simulink library "scarsLibrary"  (R2019b)
settings: Solver=VariableStepAuto  StartTime=0.0  StopTime=10.0  RelTol=1e-3
undefined symbols (not defined in the file): A_x, A_y, A_z, Actuators, added_noise, axis_switch, bb, C_d, decsec, decstart, delay, Detumbling, displacement, Earth, IAU, initDay, initEuler, initYear, linsys1, mag_sat, Magnetorquers, multiplied_noise, Re, rw, scars_library, st_freq, startTime, sun_position, t_power, WGS84
libraries: $bdroot x89, aerolibutil x15, sharedtransform x12, vrlib x9, simulink x6, aerolibtransform2 x2, aerolibgravity2 x2, aerolib6dof2 x2, simulink_extras x2, aerolibatmos2 x1, aerolibnav x1
(part 2 of 2)

== system scarsLibrary/PW-Sat2/Environment ==
  SatStates : Inport
  Atmosphere [kg/m^3] : $bdroot/Environment/Atmosphere [kg//m^3]  SystemSampleTime=-1  Latency=0  AutoFrameSizeCalculation=off
  Atmospheric Drag [N]1 : $bdroot/Environment/Atmospheric Drag [N]  SystemSampleTime=-1  Latency=0  AutoFrameSizeCalculation=off
      link override Drag [N]/Constant1: Value=area_vector
  Bus Creator : BusCreator  Inputs=4
  Gravity [N]1 : $bdroot/Environment/Gravity [N]  mass=1
  Ground : Ground
  Magnetic Field [nT]1 : $bdroot/Environment/Magnetic Field [nT]  SystemSampleTime=-1  Latency=0  AutoFrameSizeCalculation=off
  Scope : Scope
  Sum : Sum  Inputs=+|+
  Sun's Position [km]1 : $bdroot/Environment/Sun's Position [km]  SystemSampleTime=-1  Latency=0  AutoFrameSizeCalculation=off
  Env : Outport
  Forces : Outport  Port=2
  Moments : Outport  Port=3
  wires:
  Ground/1 -> Moments/1
  Atmosphere [kg/m^3]/1 -> Bus Creator/4  "Atmosphere Density [kg/m^3]"
  Gravity [N]1/1 -> Sum/2
  Bus Creator/1 -> Env/1
  Atmospheric Drag [N]1/1 -> Scope/1, Sum/1
  Magnetic Field [nT]1/1 -> Bus Creator/1  "Magnetic Field [nT]"
  Sun's Position [km]1/1 -> Bus Creator/3  "Sun's Position [km]"
  Sum/1 -> Forces/1, Bus Creator/2  "Environment Force [N]"
  SatStates/1 -> Gravity [N]1/1, Atmosphere [kg/m^3]/1, Atmospheric Drag [N]1/1, Magnetic Field [nT]1/1

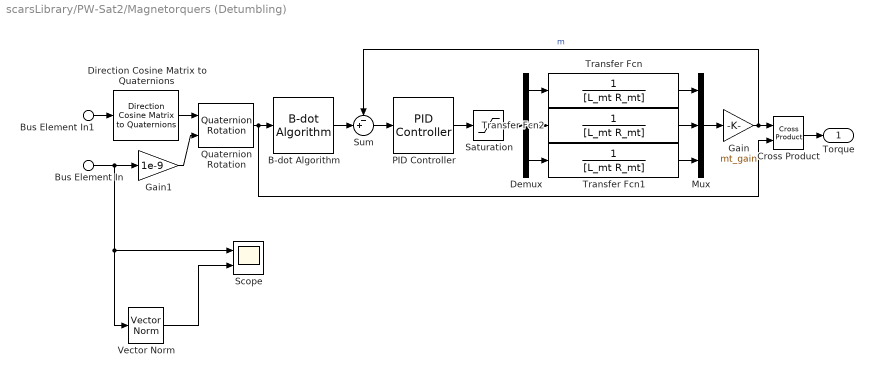
== system scarsLibrary/PW-Sat2/Magnetorquers (Detumbling) ==
  Bus Element In : Inport  PortName=Env  Element=Magnetic Field [nT]
  Bus Element In1 : Inport  Port=2  PortName=SatStates  Element=DCM_NED2B
  B-dot Algorithm : $bdroot/ Control Algorithms /B-dot Algorithm  k_gain=-0.1
  Cross Product : vrlib/Utilities/Cross Product
      settings: SourceProductName=Simulink
  Demux : Demux  Outputs=3
  Direction Cosine Matrix to Quaternions : sharedtransform/Direction Cosine Matrix  to Quaternions  aMode=0  action=None  tolerance=eps(2)
      settings: SourceProductName=Aerospace Blockset  SourceProductBaseCode=AE
  Gain : Gain  Gain=mt_gain
  Gain1 : Gain  Gain=1e-9
  Mux : Mux  Inputs=3
  PID Controller : $bdroot/ Control Algorithms /PID Controller  Kp=1  Ki=0  Kd=0  pid_sat_max=inf  pid_sat_min=-inf  pid_dz_max=0  pid_dz_min=0
  Quaternion Rotation : aerolibutil/Quaternion Rotation
  Saturation : Saturate  UpperLimit=mag_sat  LowerLimit=-mag_sat
  Scope : Scope  NumInputPorts=2
  Sum : Sum  Inputs=-+|
  Transfer Fcn : TransferFcn  Denominator=[L_mt R_mt]
  Transfer Fcn1 : TransferFcn  Denominator=[L_mt R_mt]
  Transfer Fcn2 : TransferFcn  Denominator=[L_mt R_mt]
  Vector Norm : $bdroot/Vector Norm  SystemSampleTime=-1  Latency=0  AutoFrameSizeCalculation=off
  Torque : Outport
  wires:
  Gain1/1 -> Quaternion Rotation/2
  Gain/1 -> Cross Product/1, Sum/1  "m"
  Bus Element In1/1 -> Direction Cosine Matrix to Quaternions/1
  Transfer Fcn2/1 -> Mux/2
  Cross Product/1 -> Torque/1
  Transfer Fcn1/1 -> Mux/3
  Bus Element In/1 -> Vector Norm/1, Scope/1, Gain1/1
  Transfer Fcn/1 -> Mux/1
  Demux/2 -> Transfer Fcn2/1
  Mux/1 -> Gain/1
  Quaternion Rotation/1 -> B-dot Algorithm/1, Cross Product/2
  Direction Cosine Matrix to Quaternions/1 -> Quaternion Rotation/1
  Sum/1 -> PID Controller/1
  Saturation/1 -> Demux/1
  Demux/1 -> Transfer Fcn/1
  B-dot Algorithm/1 -> Sum/2
  Demux/3 -> Transfer Fcn1/1
  PID Controller/1 -> Saturation/1
  Vector Norm/1 -> Scope/2

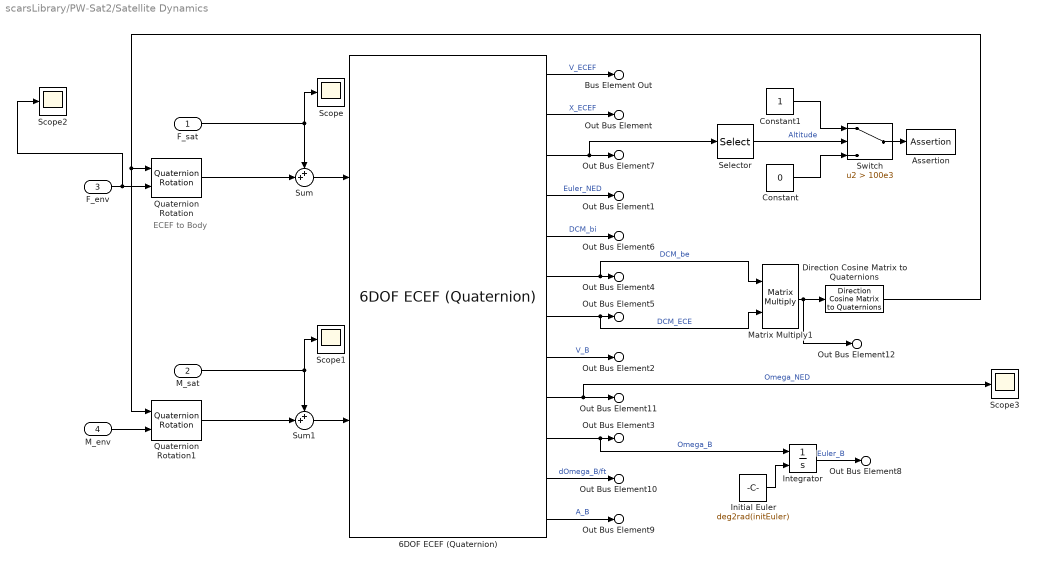
== system scarsLibrary/PW-Sat2/Satellite Dynamics ==
  note: ECEF to Body
  F_sat : Inport
  M_sat : Inport  Port=2
  F_env : Inport  Port=3
  M_env : Inport  Port=4
  6DOF ECEF (Quaternion) : aerolib6dof2/6DOF ECEF (Quaternion)  units=Metric (MKS)  mtype=Fixed  xg_0=r_lla  Vm_0=v_b  eul_0=deg2rad(initEuler)  pm_0=[0.1 0.2 0.3]  mass_0=1  mass_e=0.5  mass_f=2.0  inertia=eye(3)  inertia_e=eye(3)  inertia_f=2*eye(3)  vre_flag=on  abi_flag=off  ptype=Earth (WGS84)  R=6378137  F=1/298.257223563  w_E=7292115e-11  angle_in=Internal  LG0=0  quat_statename=''  pm_statename=''  Vm_statename=''  posECEF_statename=''  posECI_statename=''  LG_statename=''  mass_statename=''
      settings: SourceProductName=Aerospace Blockset  SourceProductBaseCode=AE
  Assertion : Assertion
  Constant : Constant  Value=0
  Constant1 : Constant
  Direction Cosine Matrix to Quaternions : sharedtransform/Direction Cosine Matrix  to Quaternions  aMode=0  action=None  tolerance=eps(2)
      settings: SourceProductName=Aerospace Blockset  SourceProductBaseCode=AE
  Initial Euler : Constant  Value=deg2rad(initEuler)
  Integrator : Integrator  InitialConditionSource=external  WrapState=on
  Matrix Multiply1 : Product  Multiplication=Matrix(*)
  Quaternion Rotation : aerolibutil/Quaternion Rotation
  Quaternion Rotation1 : aerolibutil/Quaternion Rotation
  Scope{,1..3} (4 alike) : Scope
  Selector : Selector  InputPortWidth=3  IndexOptions=Index vector (dialog)  Indices=3  OutputSizes=1
  Sum : Sum  Inputs=++|
  Sum1 : Sum  Inputs=++|
  Switch : Switch  Criteria=u2 > Threshold  Threshold=100e3
  Bus Element Out : Outport  PortName=SatStates  Element=V_ECEF
  Out Bus Element : Outport  PortName=SatStates  Element=X_ECEF
  Out Bus Element1 : Outport  PortName=SatStates  Element=Euler_NED
  Out Bus Element2 : Outport  PortName=SatStates  Element=V_B
  Out Bus Element3 : Outport  PortName=SatStates  Element=Omega_B
  Out Bus Element6 : Outport  PortName=SatStates  Element=DCM_ECI2B
  Out Bus Element4 : Outport  PortName=SatStates  Element=DCM_NED2B
  Out Bus Element5 : Outport  PortName=SatStates  Element=DCM_ECEF2NED
  Out Bus Element7 : Outport  PortName=SatStates  Element=lla
  Out Bus Element8 : Outport  PortName=SatStates  Element=Euler_B
  Out Bus Element9 : Outport  PortName=SatStates  Element=A_B
  Out Bus Element10 : Outport  PortName=SatStates  Element=dOmega_B/dt
  Out Bus Element11 : Outport  PortName=SatStates  Element=Omega_NED
  Out Bus Element12 : Outport  PortName=SatStates  Element=DCM_ECEF2B
  wires:
  Constant/1 -> Switch/3
  6DOF ECEF (Quaternion)/9 -> Scope3/1, Out Bus Element11/1  "Omega_NED"
  Initial Euler/1 -> Integrator/2
  M_env/1 -> Quaternion Rotation1/2
  6DOF ECEF (Quaternion)/12 -> Out Bus Element9/1  "A_B"
  6DOF ECEF (Quaternion)/7 -> Matrix Multiply1/2, Out Bus Element5/1  "DCM_ECE"
  6DOF ECEF (Quaternion)/11 -> Out Bus Element10/1  "dOmega_B/ft"
  6DOF ECEF (Quaternion)/3 -> Selector/1, Out Bus Element7/1
  6DOF ECEF (Quaternion)/5 -> Out Bus Element6/1  "DCM_bi"
  Sum/1 -> 6DOF ECEF (Quaternion)/1
  Integrator/1 -> Out Bus Element8/1  "Euler_B"
  Direction Cosine Matrix to Quaternions/1 -> Quaternion Rotation1/1, Quaternion Rotation/1
  F_sat/1 -> Scope/1, Sum/1
  Quaternion Rotation/1 -> Sum/2
  Quaternion Rotation1/1 -> Sum1/2
  Sum1/1 -> 6DOF ECEF (Quaternion)/2
  Matrix Multiply1/1 -> Direction Cosine Matrix to Quaternions/1, Out Bus Element12/1
  6DOF ECEF (Quaternion)/1 -> Bus Element Out/1  "V_ECEF"
  Selector/1 -> Switch/2  "Altitude"
  6DOF ECEF (Quaternion)/4 -> Out Bus Element1/1  "Euler_NED"
  6DOF ECEF (Quaternion)/6 -> Matrix Multiply1/1, Out Bus Element4/1  "DCM_be"
  6DOF ECEF (Quaternion)/2 -> Out Bus Element/1  "X_ECEF"
  Switch/1 -> Assertion/1
  Constant1/1 -> Switch/1
  6DOF ECEF (Quaternion)/10 -> Integrator/1, Out Bus Element3/1  "Omega_B"
  6DOF ECEF (Quaternion)/8 -> Out Bus Element2/1  "V_B"
  M_sat/1 -> Sum1/1, Scope1/1
  F_env/1 -> Scope2/1, Quaternion Rotation/2

== system scarsLibrary/Sensors/Accelerometer ==
  SatStates : Inport
  Bus Element In : Inport  Port=2  PortName=Env  Element=Gravitational Force [N]
  Bus Selector : BusSelector  OutputSignals=A_B,Omega_B,dOmega_B/dt
  Constant : Constant  Value=[0 0 0]
  Three-axis Accelerometer : aerolibnav/Three-axis Accelerometer  units=Metric (MKS)  acc=acc  gtype=on  dtype_a=on  w_a=w_a  z_a=z_a  a_sf_cc=[1 0 0; 0 1 0; 0 0 1]  a_bias=a_bias*[1 1 1]  a_Ts=0  a_rand=on  a_seeds=[23093 23094 23095]  a_pow=a_pow*[1 1 1]  a_sat="[-a_min  -a_min  -a_min a_max a_max a_max]"
      settings: SourceProductName=Aerospace Blockset  SourceProductBaseCode=AE
  Zero-Order Hold : ZeroOrderHold  SampleTime=1/freq
  A_B : Outport
  wires:
  SatStates/1 -> Bus Selector/1
  Constant/1 -> Three-axis Accelerometer/4
  Bus Selector/1 -> Three-axis Accelerometer/1  "<A_B>"
  Bus Selector/2 -> Three-axis Accelerometer/2  "<Omega_B>"
  Bus Selector/3 -> Three-axis Accelerometer/3  "<dOmega_B/dt>"
  Bus Element In/1 -> Three-axis Accelerometer/5
  Three-axis Accelerometer/1 -> Zero-Order Hold/1
  Zero-Order Hold/1 -> A_B/1

== system scarsLibrary/Sensors/Earth- & Sun-sensor ==
  Bus Element In1 : Inport  PortName=SatStates  Element=X_ECEF
  Bus Element In : Inport  Port=2  PortName=Env  Element=Sun's Position [km]
  Euler_B : Outport
  wires:
  Bus Element In/1 -> Euler_B/1

== system scarsLibrary/Sensors/GPS Receiver ==
  Bus Element In : Inport  PortName=SatStates  Element=X_ECEF
  X_ECEF : Outport
  wires:
  Bus Element In/1 -> X_ECEF/1

== system scarsLibrary/Sensors/Gyros ==
  note: noise_power  = [0.1]
      | sample_time = 0.1
  note: wn = 1000*2*pi; % natural frequency [not in Hz, but can be transferred] dynamics rad/s
      | w = 12.5*2*pi; % cutoff frequency [Hz*2pi = deg/s] LPF rad/s
      | zeta = sqrt(2)/2; % damping ratio
      | z = zeta; %?
  Bus Element In : Inport  PortName=SatStates  Element=Omega_B
  Add : Sum
  Add1 : Sum
  Band-Limited White Noise : simulink/Sources/Band-Limited White Noise  Cov=[g_power]  Ts=1/g_freq  seed=[23341]
  Constant : Constant  Value=g_bias
  Demux : Demux  Outputs=3
  Mux : Mux  Inputs=3
  Transfer Fcn : TransferFcn  Numerator=[g_wn^2]  Denominator=[1 2*g_zeta*(g_wn) (g_wn)^2]
  Transfer Fcn1 : TransferFcn  Numerator=[g_wn^2]  Denominator=[1 2*g_zeta*(g_wn) (g_wn)^2]
  Transfer Fcn2 : TransferFcn  Numerator=[g_wn^2]  Denominator=[1 2*g_zeta*(g_wn) (g_wn)^2]
  Zero-Order Hold : ZeroOrderHold  SampleTime=1/g_freq
  Omega_B : Outport
  wires:
  Constant/1 -> Add/2
  Add/1 -> Add1/1
  Band-Limited White Noise/1 -> Add1/2
  Add1/1 -> Zero-Order Hold/1
  Zero-Order Hold/1 -> Omega_B/1
  Bus Element In/1 -> Demux/1
  Demux/2 -> Transfer Fcn/1
  Demux/1 -> Transfer Fcn1/1
  Demux/3 -> Transfer Fcn2/1
  Transfer Fcn/1 -> Mux/2
  Transfer Fcn1/1 -> Mux/1
  Transfer Fcn2/1 -> Mux/3
  Mux/1 -> Add/1

== system scarsLibrary/Sensors/Ideal Angle ==
  Bus Element In : Inport  PortName=SatStates  Element=Euler_B
  Euler_B : Outport
  wires:
  Bus Element In/1 -> Euler_B/1

== system scarsLibrary/Sensors/Ideal Position ==
  Bus Element In : Inport  PortName=SatStates  Element=X_ECEF
  X_ECEF : Outport
  wires:
  Bus Element In/1 -> X_ECEF/1

== system scarsLibrary/Sensors/Ideal Rate ==
  Bus Element In : Inport  PortName=SatStates  Element=Euler_B
  Omega_B : Outport
  wires:
  Bus Element In/1 -> Omega_B/1

== system scarsLibrary/Sensors/Magnetometer ==
  Bus Element In : Inport  PortName=Env  Element=Magnetic Field [nT]
  Bias : Constant  Value=m_bias
  Noise : simulink/Sources/Band-Limited White Noise  Cov=m_power*[1 1 1]  Ts=1/m_freq  seed="[ randi(1000, 1, 3)  ]"
  Sum1 : Sum  Inputs=+++
  "Zero-Order Hold " : ZeroOrderHold  SampleTime=1/m_freq
  B : Outport
  wires:
  Bias/1 -> Sum1/3
  Bus Element In/1 -> Sum1/2
  "Zero-Order Hold "/1 -> B/1
  Noise/1 -> Sum1/1
  Sum1/1 -> "Zero-Order Hold "/1

== system scarsLibrary/Sensors/Simple Angle ==
  Bus Element In : Inport  PortName=SatStates  Element=Euler_B
  Euler_B : Outport
  wires:
  Bus Element In/1 -> Euler_B/1

== system scarsLibrary/Sensors/Simple Position ==
  Bus Element In : Inport  PortName=SatStates  Element=X_ECEF
  X_ECEF : Outport
  wires:
  Bus Element In/1 -> X_ECEF/1

== system scarsLibrary/Sensors/Simple Rate ==
  Bus Element In : Inport  PortName=SatStates  Element=Euler_B
  Omega_B : Outport
  wires:
  Bus Element In/1 -> Omega_B/1

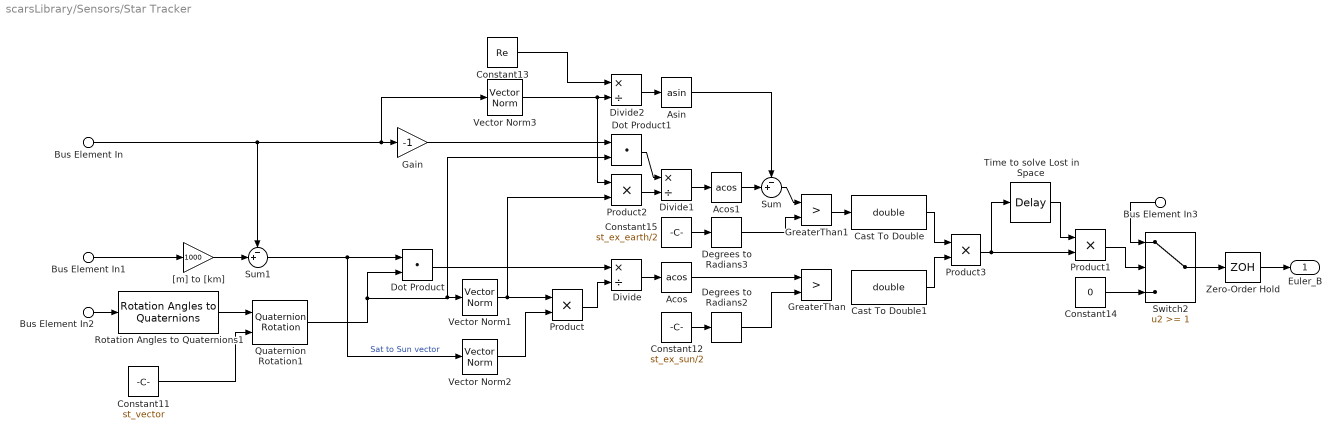
== system scarsLibrary/Sensors/Star Tracker ==
  Bus Element In : Inport  PortName=SatStates  Element=X_ECEF
  Bus Element In2 : Inport  PortName=SatStates  Element=Euler_B
  Bus Element In3 : Inport  PortName=SatStates  Element=Euler_B
  Bus Element In1 : Inport  Port=2  PortName=Env  Element=Sun's Position [km]
  Acos : Trigonometry  Operator=acos
  Acos1 : Trigonometry  Operator=acos
  Asin : Trigonometry  Operator=asin
  Cast To Double : DataTypeConversion  OutDataTypeStr=double
  Cast To Double1 : DataTypeConversion  OutDataTypeStr=double
  Constant11 : Constant  Value=st_vector
  Constant12 : Constant  Value=st_ex_sun/2
  Constant13 : Constant  Value=Re
  Constant14 : Constant  Value=0
  Constant15 : Constant  Value=st_ex_earth/2
  Degrees to Radians2 : simulink_extras/Transformations/Degrees to Radians
  Degrees to Radians3 : simulink_extras/Transformations/Degrees to Radians
  Divide : Product  Inputs=*/
  Divide1 : Product  Inputs=*/
  Divide2 : Product  Inputs=*/
  Dot Product : DotProduct  InputSameDT=on  OutDataTypeStr=Inherit: Inherit via internal rule
  Dot Product1 : DotProduct  InputSameDT=on  OutDataTypeStr=Inherit: Inherit via internal rule
  Gain : Gain  Gain=-1
  GreaterThan : RelationalOperator  Operator=>  OutDataTypeStr=boolean  RndMeth=Simplest
  GreaterThan1 : RelationalOperator  Operator=>  OutDataTypeStr=boolean  RndMeth=Simplest
  Product{,1..3} (4 alike) : Product
  Quaternion Rotation1 : aerolibutil/Quaternion Rotation
  Rotation Angles to Quaternions1 : sharedtransform/Rotation Angles to Quaternions  rotationOrder=XYZ  aMode=aMode
      settings: SourceProductName=Aerospace Blockset  SourceProductBaseCode=AE
  Sum : Sum  Inputs=-+|
  Sum1 : Sum  Inputs=-+|
  Switch2 : Switch  Threshold=1
  Time to solve Lost in Space : TransportDelay  DelayTime=st_lost  InitialOutput=1
  Vector Norm1 : $bdroot/Vector Norm  SystemSampleTime=-1  Latency=0  AutoFrameSizeCalculation=off
  Vector Norm2 : $bdroot/Vector Norm  SystemSampleTime=-1  Latency=0  AutoFrameSizeCalculation=off
  Vector Norm3 : $bdroot/Vector Norm  SystemSampleTime=-1  Latency=0  AutoFrameSizeCalculation=off
  Zero-Order Hold : ZeroOrderHold  SampleTime=1/st_freq
  "[m] to [km]" : Gain  Gain=1000
  Euler_B : Outport
  wires:
  Rotation Angles to Quaternions1/1 -> Quaternion Rotation1/1
  Bus Element In/1 -> Sum1/1, Vector Norm3/1, Gain/1
  Acos/1 -> GreaterThan/1
  Constant13/1 -> Divide2/1
  "[m] to [km]"/1 -> Sum1/2
  Quaternion Rotation1/1 -> Dot Product/2, Dot Product1/2, Vector Norm1/1
  Vector Norm1/1 -> Product2/2, Product/1
  Product/1 -> Divide/2
  Switch2/1 -> Zero-Order Hold/1
  Bus Element In2/1 -> Rotation Angles to Quaternions1/1
  Product1/1 -> Switch2/2
  Product3/1 -> Time to solve Lost in Space/1, Product1/2
  Constant15/1 -> Degrees to Radians3/1
  Degrees to Radians3/1 -> GreaterThan1/2
  Constant14/1 -> Switch2/3
  Vector Norm3/1 -> Product2/1, Divide2/2
  Time to solve Lost in Space/1 -> Product1/1
  Sum1/1 -> Vector Norm2/1, Dot Product/1  "Sat to Sun vector"
  Degrees to Radians2/1 -> GreaterThan/2
  Product2/1 -> Divide1/2
  Dot Product/1 -> Divide/1
  Constant11/1 -> Quaternion Rotation1/2
  Divide2/1 -> Asin/1
  Bus Element In3/1 -> Switch2/1
  Constant12/1 -> Degrees to Radians2/1
  Dot Product1/1 -> Divide1/1
  Gain/1 -> Dot Product1/1
  Divide1/1 -> Acos1/1
  Divide/1 -> Acos/1
  Bus Element In1/1 -> "[m] to [km]"/1
  Vector Norm2/1 -> Product/2
  Acos1/1 -> Sum/2
  Sum/1 -> GreaterThan1/1
  Asin/1 -> Sum/1
  Zero-Order Hold/1 -> Euler_B/1
  GreaterThan1/1 -> Cast To Double/1
  Cast To Double1/1 -> Product3/2
  Cast To Double/1 -> Product3/1

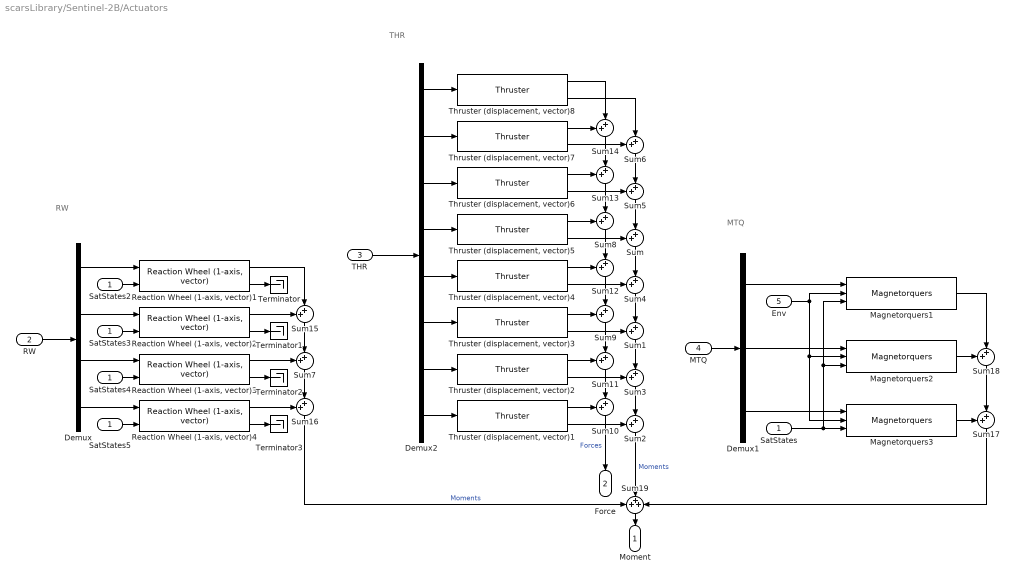
== system scarsLibrary/Sentinel-2B/Actuators ==
  note: MTQ
  note: RW
  note: THR
  SatStates : Inport
  RW : Inport  Port=2
  THR : Inport  Port=3
  MTQ : Inport  Port=4
  Env : Inport  Port=5
  Demux : Demux
  Demux1 : Demux  Outputs=3
  Demux2 : Demux  Outputs=8
  Magnetorquers1 : $bdroot/Actuators/Magnetorquers  L_mt=2.666  R_mt=3.621  l_c_mt=0.25  w_c_mt=7.965e-3  d_w_mt=4.04e-4  mag_vol_max=3  mag_vol_min=-3
  Magnetorquers2 : $bdroot/Actuators/Magnetorquers  L_mt=2.666  R_mt=3.621  l_c_mt=0.25  w_c_mt=7.965e-3  d_w_mt=4.04e-4  mag_vol_max=3  mag_vol_min=-3
  Magnetorquers3 : $bdroot/Actuators/Magnetorquers  L_mt=2.666  R_mt=3.621  l_c_mt=0.25  w_c_mt=7.965e-3  d_w_mt=4.04e-4  mag_vol_max=3  mag_vol_min=-3
  Reaction Wheel (1-axis, vector){1..4} (4 alike) : $bdroot/Actuators/Reaction Wheel (1-axis, vector)  op_vect=[1 1 1]  N=25e-3  R=0.1  J=1  c=0.0001  vel_max=6000*2*pi/60  torq_max=1.5e-3  i_max=0.5  rw_power=0.0001  rw_freq=0.1
  SatStates{2..5} (4 alike) : InportShadow
  Sum{,1..18} (19 alike) : Sum  Inputs=++|
  Sum19 : Sum  Inputs=+++
  Terminator{,1..3} (4 alike) : Terminator
  Thruster (displacement, vector){1..8} (8 alike) : $bdroot/Actuators/Thruster  SystemSampleTime=-1  Latency=0  AutoFrameSizeCalculation=off
  Moment : Outport
  Force : Outport  Port=2
  wires:
  Demux2/1 -> "Thruster (displacement, vector)8"/1
  "Reaction Wheel (1-axis, vector)4"/1 -> Sum16/1
  Sum15/1 -> Sum7/2
  Demux/4 -> "Reaction Wheel (1-axis, vector)4"/1
  "Thruster (displacement, vector)2"/2 -> Sum3/1
  "Thruster (displacement, vector)2"/1 -> Sum11/1
  "Thruster (displacement, vector)3"/2 -> Sum1/1
  Sum6/1 -> Sum5/2
  "Thruster (displacement, vector)6"/2 -> Sum5/1
  "Reaction Wheel (1-axis, vector)4"/2 -> Terminator3/1
  Demux2/3 -> "Thruster (displacement, vector)6"/1
  Sum13/1 -> Sum8/2
  Demux1/3 -> Magnetorquers3/1
  Sum11/1 -> Sum10/2
  Sum14/1 -> Sum13/2
  "Thruster (displacement, vector)7"/2 -> Sum6/1
  Sum/1 -> Sum4/2
  Sum9/1 -> Sum11/2
  Sum8/1 -> Sum12/2
  "Thruster (displacement, vector)7"/1 -> Sum14/1
  Demux1/2 -> Magnetorquers2/1
  Sum2/1 -> Sum19/2  "Moments"
  Demux2/5 -> "Thruster (displacement, vector)4"/1
  Demux1/1 -> Magnetorquers1/1
  "Thruster (displacement, vector)4"/2 -> Sum4/1
  Sum4/1 -> Sum1/2
  "Reaction Wheel (1-axis, vector)2"/1 -> Sum15/1
  Env/1 -> Magnetorquers1/2, Magnetorquers3/2, Magnetorquers2/2
  Demux/2 -> "Reaction Wheel (1-axis, vector)2"/1
  Sum10/1 -> Force/1  "Forces"
  Sum16/1 -> Sum19/1  "Moments"
  Demux2/2 -> "Thruster (displacement, vector)7"/1
  SatStates/1 -> Magnetorquers1/3, Magnetorquers2/3, Magnetorquers3/3
  "Reaction Wheel (1-axis, vector)1"/2 -> Terminator/1
  "Reaction Wheel (1-axis, vector)3"/2 -> Terminator2/1
  Sum5/1 -> Sum/2
  "Reaction Wheel (1-axis, vector)2"/2 -> Terminator1/1
  Demux2/8 -> "Thruster (displacement, vector)1"/1
  "Thruster (displacement, vector)8"/2 -> Sum6/2
  SatStates3/1 -> "Reaction Wheel (1-axis, vector)2"/2
  SatStates5/1 -> "Reaction Wheel (1-axis, vector)4"/2
  Demux/3 -> "Reaction Wheel (1-axis, vector)3"/1
  SatStates4/1 -> "Reaction Wheel (1-axis, vector)3"/2
  Demux2/7 -> "Thruster (displacement, vector)2"/1
  Demux2/6 -> "Thruster (displacement, vector)3"/1
  Demux/1 -> "Reaction Wheel (1-axis, vector)1"/1
  Sum1/1 -> Sum3/2
  "Reaction Wheel (1-axis, vector)1"/1 -> Sum15/2
  "Thruster (displacement, vector)4"/1 -> Sum12/1
  Demux2/4 -> "Thruster (displacement, vector)5"/1
  Sum7/1 -> Sum16/2
  "Thruster (displacement, vector)6"/1 -> Sum13/1
  "Thruster (displacement, vector)1"/2 -> Sum2/1
  "Thruster (displacement, vector)1"/1 -> Sum10/1
  "Thruster (displacement, vector)5"/2 -> Sum/1
  Sum3/1 -> Sum2/2
  "Reaction Wheel (1-axis, vector)3"/1 -> Sum7/1
  SatStates2/1 -> "Reaction Wheel (1-axis, vector)1"/2
  "Thruster (displacement, vector)5"/1 -> Sum8/1
  "Thruster (displacement, vector)8"/1 -> Sum14/2
  Sum12/1 -> Sum9/2
  "Thruster (displacement, vector)3"/1 -> Sum9/1
  Sum18/1 -> Sum17/2
  Sum17/1 -> Sum19/3
  Magnetorquers1/1 -> Sum18/2
  Magnetorquers2/1 -> Sum18/1
  Magnetorquers3/1 -> Sum17/1
  Sum19/1 -> Moment/1
  RW/1 -> Demux/1
  THR/1 -> Demux2/1
  MTQ/1 -> Demux1/1

== system scarsLibrary/Sentinel-2B/OBC ==
  Sensors : Inport
  Ground : Ground
  Ground1 : Ground
  Ground2 : Ground
  Terminator : Terminator
  RW : Outport
  THR : Outport  Port=2
  MTQ : Outport  Port=3
  wires:
  Sensors/1 -> Terminator/1
  Ground/1 -> RW/1
  Ground1/1 -> THR/1
  Ground2/1 -> MTQ/1

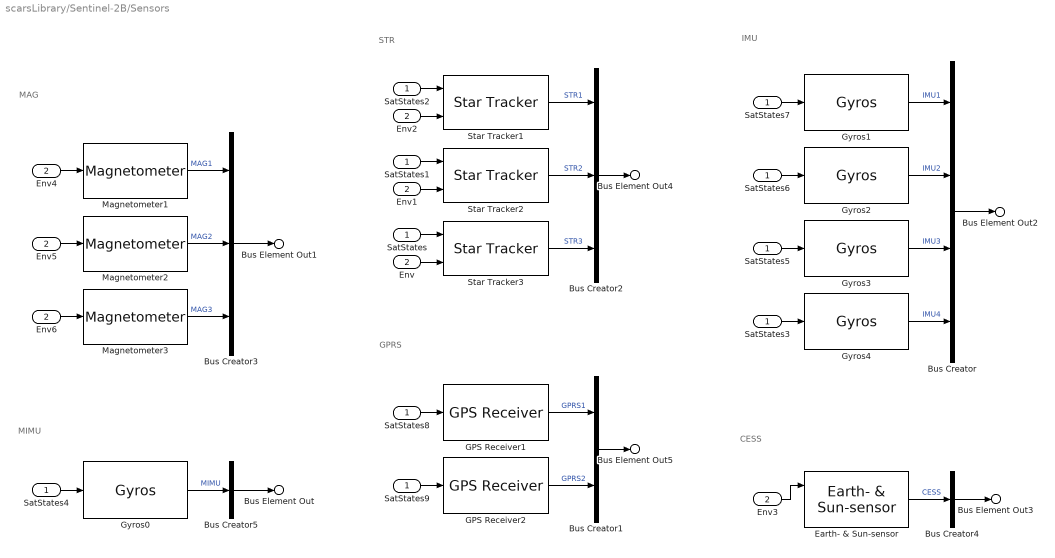
== system scarsLibrary/Sentinel-2B/Sensors ==
  note: MIMU
  note: MAG
  note: CESS
  note: IMU
  note: GPRS
  note: STR
  "SatStates " : Inport
  "Env " : Inport  Port=2
  Bus Creator : BusCreator  Inputs=4
  Bus Creator1 : BusCreator  Inputs=2
  Bus Creator2 : BusCreator  Inputs=3
  Bus Creator3 : BusCreator  Inputs=3
  Bus Creator4 : BusCreator  Inputs=1
  Bus Creator5 : BusCreator  Inputs=1
  Earth- & Sun-sensor : $bdroot/Sensors/Earth- & Sun-sensor  SystemSampleTime=-1  Latency=0  AutoFrameSizeCalculation=off
  Env{1..6} (6 alike) : InportShadow  Port=2
  GPS Receiver1 : $bdroot/Sensors/GPS Receiver  SystemSampleTime=-1  Latency=0  AutoFrameSizeCalculation=off
  GPS Receiver2 : $bdroot/Sensors/GPS Receiver  SystemSampleTime=-1  Latency=0  AutoFrameSizeCalculation=off
  Gyros{0..4} (5 alike) : $bdroot/Sensors/Gyros  g_wn=1000*2*pi  g_zeta=sqrt(2)/2  g_freq=80  g_bias=0  g_power=(0.04)^2  g_max=deg2rad(100)  g_min=-deg2rad(100)
  Magnetometer1 : $bdroot/Sensors/Magnetometer  m_power=0.1  m_freq=10  m_bias=[0.01 0.01 0.01]
  Magnetometer2 : $bdroot/Sensors/Magnetometer  m_power=0.1  m_freq=10  m_bias=[0.01 0.01 0.01]
  Magnetometer3 : $bdroot/Sensors/Magnetometer  m_power=0.1  m_freq=10  m_bias=[0.01 0.01 0.01]
  SatStates{1..9} (9 alike) : InportShadow
  Star Tracker1 : $bdroot/Sensors/Star Tracker  st_vector=[0 0 -1]  st_ex_sun=20  st_ex_earth=20  st_lost=5  Parameter5=10
  Star Tracker2 : $bdroot/Sensors/Star Tracker  st_vector=[0 0 -1]  st_ex_sun=20  st_ex_earth=20  st_lost=5  Parameter5=10
  Star Tracker3 : $bdroot/Sensors/Star Tracker  st_vector=[0 0 -1]  st_ex_sun=20  st_ex_earth=20  st_lost=5  Parameter5=10
  Bus Element Out : Outport  PortName=Sensors  Element=MIMU
  Bus Element Out1 : Outport  PortName=Sensors  Element=MAG
  Bus Element Out2 : Outport  PortName=Sensors  Element=IMU
  Bus Element Out3 : Outport  PortName=Sensors  Element=CESS
  Bus Element Out4 : Outport  PortName=Sensors  Element=STR
  Bus Element Out5 : Outport  PortName=Sensors  Element=GPRS
  wires:
  Env1/1 -> Star Tracker2/2
  Star Tracker1/1 -> Bus Creator2/1  "STR1"
  SatStates1/1 -> Star Tracker2/1
  Star Tracker2/1 -> Bus Creator2/2  "STR2"
  Env2/1 -> Star Tracker1/2
  "Env "/1 -> Star Tracker3/2
  "SatStates "/1 -> Star Tracker3/1
  Star Tracker3/1 -> Bus Creator2/3  "STR3"
  SatStates2/1 -> Star Tracker1/1
  Env5/1 -> Magnetometer2/1
  Env4/1 -> Magnetometer1/1
  Magnetometer1/1 -> Bus Creator3/1  "MAG1"
  Env6/1 -> Magnetometer3/1
  Magnetometer2/1 -> Bus Creator3/2  "MAG2"
  SatStates8/1 -> GPS Receiver1/1
  Env3/1 -> Earth- & Sun-sensor/1
  SatStates9/1 -> GPS Receiver2/1
  GPS Receiver2/1 -> Bus Creator1/2  "GPRS2"
  Magnetometer3/1 -> Bus Creator3/3  "MAG3"
  Earth- & Sun-sensor/1 -> Bus Creator4/1  "CESS"
  GPS Receiver1/1 -> Bus Creator1/1  "GPRS1"
  SatStates3/1 -> Gyros4/1
  Gyros3/1 -> Bus Creator/3  "IMU3"
  Gyros4/1 -> Bus Creator/4  "IMU4"
  Gyros1/1 -> Bus Creator/1  "IMU1"
  Gyros2/1 -> Bus Creator/2  "IMU2"
  SatStates4/1 -> Gyros0/1
  Gyros0/1 -> Bus Creator5/1  "MIMU"
  SatStates6/1 -> Gyros2/1
  SatStates7/1 -> Gyros1/1
  SatStates5/1 -> Gyros3/1
  Bus Creator5/1 -> Bus Element Out/1
  Bus Creator3/1 -> Bus Element Out1/1
  Bus Creator/1 -> Bus Element Out2/1
  Bus Creator4/1 -> Bus Element Out3/1
  Bus Creator2/1 -> Bus Element Out4/1
  Bus Creator1/1 -> Bus Element Out5/1

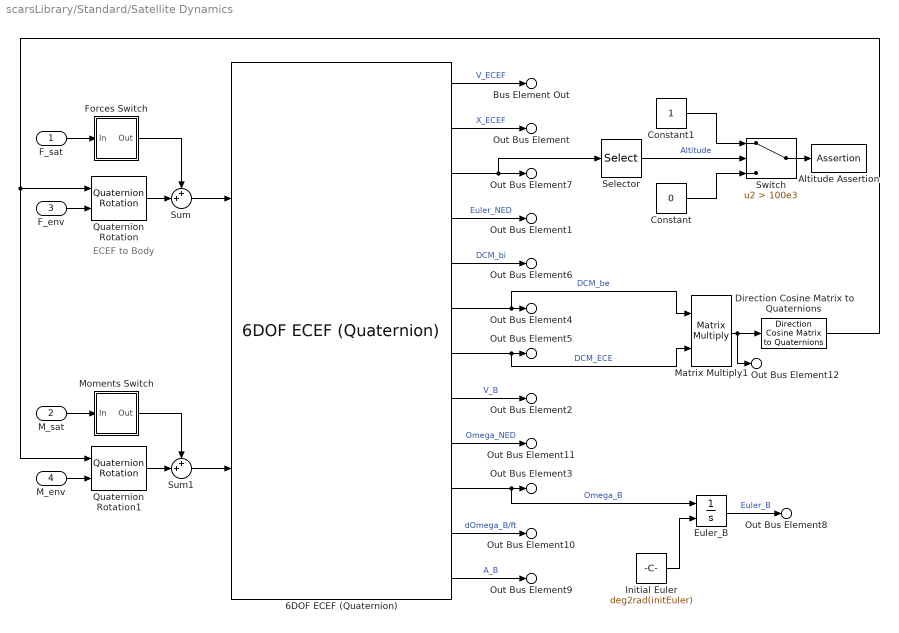
== system scarsLibrary/Standard/Satellite Dynamics ==
  note: ECEF to Body
  F_sat : Inport
  M_sat : Inport  Port=2
  F_env : Inport  Port=3
  M_env : Inport  Port=4
  6DOF ECEF (Quaternion) : aerolib6dof2/6DOF ECEF (Quaternion)  units=Metric (MKS)  mtype=Fixed  xg_0=r_lla  Vm_0=v_b  eul_0=deg2rad(initEuler)  pm_0=deg2rad(initEulerRates)  mass_0=mass  mass_e=0.5  mass_f=2.0  inertia=eye(3)  inertia_e=eye(3)  inertia_f=2*eye(3)  vre_flag=on  abi_flag=off  ptype=Earth (WGS84)  R=6378137  F=1/298.257223563  w_E=7292115e-11  angle_in=Internal  LG0=0  quat_statename=''  pm_statename=''  Vm_statename=''  posECEF_statename=''  posECI_statename=''  LG_statename=''  mass_statename=''
      settings: SourceProductName=Aerospace Blockset  SourceProductBaseCode=AE
  Altitude Assertion : Assertion
  Constant : Constant  Value=0
  Constant1 : Constant
  Direction Cosine Matrix to Quaternions : sharedtransform/Direction Cosine Matrix  to Quaternions  aMode=0  action=None  tolerance=eps(2)
      settings: SourceProductName=Aerospace Blockset  SourceProductBaseCode=AE
  Euler_B : Integrator  InitialConditionSource=external  WrapState=on
  Forces Switch : Subsystem
  Initial Euler : Constant  Value=deg2rad(initEuler)
  Matrix Multiply1 : Product  Multiplication=Matrix(*)
  Moments Switch : Subsystem
  Quaternion Rotation : aerolibutil/Quaternion Rotation
  Quaternion Rotation1 : aerolibutil/Quaternion Rotation
  Selector : Selector  InputPortWidth=3  IndexOptions=Index vector (dialog)  Indices=3  OutputSizes=1
  Sum : Sum  Inputs=++|
  Sum1 : Sum  Inputs=++|
  Switch : Switch  Criteria=u2 > Threshold  Threshold=100e3
  Bus Element Out : Outport  PortName=SatStates  Element=V_ECEF
  Out Bus Element : Outport  PortName=SatStates  Element=X_ECEF
  Out Bus Element1 : Outport  PortName=SatStates  Element=Euler_NED
  Out Bus Element2 : Outport  PortName=SatStates  Element=V_B
  Out Bus Element3 : Outport  PortName=SatStates  Element=Omega_B
  Out Bus Element6 : Outport  PortName=SatStates  Element=DCM_ECI2B
  Out Bus Element4 : Outport  PortName=SatStates  Element=DCM_NED2B
  Out Bus Element5 : Outport  PortName=SatStates  Element=DCM_ECEF2NED
  Out Bus Element7 : Outport  PortName=SatStates  Element=lla
  Out Bus Element8 : Outport  PortName=SatStates  Element=Euler_B
  Out Bus Element9 : Outport  PortName=SatStates  Element=A_B
  Out Bus Element10 : Outport  PortName=SatStates  Element=dOmega_B/dt
  Out Bus Element11 : Outport  PortName=SatStates  Element=Omega_NED
  Out Bus Element12 : Outport  PortName=SatStates  Element=DCM_ECEF2B
  wires:
  6DOF ECEF (Quaternion)/1 -> Bus Element Out/1  "V_ECEF"
  6DOF ECEF (Quaternion)/8 -> Out Bus Element2/1  "V_B"
  6DOF ECEF (Quaternion)/2 -> Out Bus Element/1  "X_ECEF"
  6DOF ECEF (Quaternion)/6 -> Matrix Multiply1/1, Out Bus Element4/1  "DCM_be"
  6DOF ECEF (Quaternion)/7 -> Matrix Multiply1/2, Out Bus Element5/1  "DCM_ECE"
  6DOF ECEF (Quaternion)/4 -> Out Bus Element1/1  "Euler_NED"
  6DOF ECEF (Quaternion)/10 -> Euler_B/1, Out Bus Element3/1  "Omega_B"
  Quaternion Rotation1/1 -> Sum1/2
  Sum1/1 -> 6DOF ECEF (Quaternion)/2
  Matrix Multiply1/1 -> Direction Cosine Matrix to Quaternions/1, Out Bus Element12/1
  F_sat/1 -> Forces Switch/1(In)
  Quaternion Rotation/1 -> Sum/2
  F_env/1 -> Quaternion Rotation/2
  Direction Cosine Matrix to Quaternions/1 -> Quaternion Rotation1/1, Quaternion Rotation/1
  Forces Switch/1(Out) -> Sum/1
  M_sat/1 -> Moments Switch/1(In)
  Moments Switch/1(Out) -> Sum1/1
  6DOF ECEF (Quaternion)/5 -> Out Bus Element6/1  "DCM_bi"
  6DOF ECEF (Quaternion)/9 -> Out Bus Element11/1  "Omega_NED"
  6DOF ECEF (Quaternion)/11 -> Out Bus Element10/1  "dOmega_B/ft"
  6DOF ECEF (Quaternion)/12 -> Out Bus Element9/1  "A_B"
  Sum/1 -> 6DOF ECEF (Quaternion)/1
  M_env/1 -> Quaternion Rotation1/2
  Initial Euler/1 -> Euler_B/2
  Euler_B/1 -> Out Bus Element8/1  "Euler_B"
  Selector/1 -> Switch/2  "Altitude"
  Switch/1 -> Altitude Assertion/1
  6DOF ECEF (Quaternion)/3 -> Selector/1, Out Bus Element7/1
  Constant/1 -> Switch/3
  Constant1/1 -> Switch/1

== system scarsLibrary/Variants/Subsystem ==
  In1 : Inport
  In2 : Inport  Port=2
  In3 : Inport  Port=3
  In4 : Inport  Port=4
  Gravity [N] : $bdroot/Environment/Gravity [N]  mass=0
  Satellite Dynamics1 : $bdroot/Advanced/Satellite Dynamics  Parameter4=Keplerian Elements  epoch=0  mass=0  a=6356e3+400e3  e=0  incl=0  RA=0  w=0  TA=0  initEuler=[0 0 0]  initEulerRates=[0 0 0]  TA_copy=0  TA_copy_copy=0  TA_copy_copy_copy=[10 25]  TA_copy_copy_copy_copy=[10 25]  initEuler_copy=[0 0 0]  initEulerRates_copy=[0 0 0]
  Out1 : Outport
  wires:
  In3/1 -> Satellite Dynamics1/3
  Satellite Dynamics1/1 -> Out1/1
  In4/1 -> Satellite Dynamics1/4
  In1/1 -> Satellite Dynamics1/1
  In2/1 -> Satellite Dynamics1/2

== system scarsLibrary/Variants/Subsystem1 ==
  In1 : Inport
  In2 : Inport  Port=2
  In3 : Inport  Port=3
  In4 : Inport  Port=4
  Gravity [N] : $bdroot/Environment/Gravity [N]  mass=0
  Satellite Dynamics1 : $bdroot/Advanced/Satellite Dynamics  Parameter4=Keplerian Elements  epoch=0  mass=0  a=6356e3+400e3  e=0  incl=0  RA=0  w=0  TA=0  initEuler=[0 0 0]  initEulerRates=[0 0 0]  TA_copy=0  TA_copy_copy=0  TA_copy_copy_copy=[10 25]  TA_copy_copy_copy_copy=[10 25]  initEuler_copy=[0 0 0]  initEulerRates_copy=[0 0 0]
  Out1 : Outport
  wires:
  In2/1 -> Satellite Dynamics1/2
  In1/1 -> Satellite Dynamics1/1
  In4/1 -> Satellite Dynamics1/4
  Satellite Dynamics1/1 -> Out1/1
  In3/1 -> Satellite Dynamics1/3

== system scarsLibrary/Variants/Subsystem2 ==
  In1 : Inport
  In2 : Inport  Port=2
  In3 : Inport  Port=3
  In4 : Inport  Port=4
  Gravity [N] : $bdroot/Environment/Gravity [N]  mass=0
  Satellite Dynamics1 : $bdroot/Advanced/Satellite Dynamics  Parameter4=Keplerian Elements  epoch=0  mass=0  a=6356e3+400e3  e=0  incl=0  RA=0  w=0  TA=0  initEuler=[0 0 0]  initEulerRates=[0 0 0]  TA_copy=0  TA_copy_copy=0  TA_copy_copy_copy=[10 25]  TA_copy_copy_copy_copy=[10 25]  initEuler_copy=[0 0 0]  initEulerRates_copy=[0 0 0]
  Out1 : Outport
  wires:
  In3/1 -> Satellite Dynamics1/3
  Satellite Dynamics1/1 -> Out1/1
  In4/1 -> Satellite Dynamics1/4
  In1/1 -> Satellite Dynamics1/1
  In2/1 -> Satellite Dynamics1/2

== system scarsLibrary/Variants/Subsystem3 ==
  In1 : Inport
  In2 : Inport  Port=2
  In3 : Inport  Port=3
  In4 : Inport  Port=4
  Gravity [N] : $bdroot/Environment/Gravity [N]  mass=0
  Satellite Dynamics1 : $bdroot/Advanced/Satellite Dynamics  Parameter4=Keplerian Elements  epoch=0  mass=0  a=6356e3+400e3  e=0  incl=0  RA=0  w=0  TA=0  initEuler=[0 0 0]  initEulerRates=[0 0 0]  TA_copy=0  TA_copy_copy=0  TA_copy_copy_copy=[10 25]  TA_copy_copy_copy_copy=[10 25]  initEuler_copy=[0 0 0]  initEulerRates_copy=[0 0 0]
  Out1 : Outport
  wires:
  In2/1 -> Satellite Dynamics1/2
  In1/1 -> Satellite Dynamics1/1
  In4/1 -> Satellite Dynamics1/4
  Satellite Dynamics1/1 -> Out1/1
  In3/1 -> Satellite Dynamics1/3

== system scarsLibrary/Virtual World/Position to VRML ==
  X_ECEF : Inport
  Demux1 : Demux  Outputs=3
  Gain3 : Gain  Gain=-1
  Mux1 : Mux  Inputs=3
  pos : Outport
  wires:
  Mux1/1 -> pos/1
  Demux1/3 -> Mux1/2
  Demux1/2 -> Mux1/3
  Demux1/1 -> Gain3/1
  X_ECEF/1 -> Demux1/1
  Gain3/1 -> Mux1/1

== system scarsLibrary/Virtual World/Quaternion to VRML ==
  q : Inport
  Acos : Trigonometry  Operator=acos
  Demux : Demux
  Gain1 : Gain  Gain=2
  Gain2 : Gain  Gain=-1
  Mux : Mux
  rot : Outport
  wires:
  Demux/4 -> Mux/1
  Acos/1 -> Gain1/1
  Gain1/1 -> Mux/4
  Demux/2 -> Mux/2
  Demux/1 -> Mux/3
  q/1 -> Demux/1
  Mux/1 -> rot/1
  Demux/3 -> Gain2/1
  Gain2/1 -> Acos/1

== system scarsLibrary/Virtual World/SCARS to VRML ==
  SatStates : Inport
  Env : Inport  Port=2
  Bus Selector : BusSelector  OutputSignals=q_ECEF2Body,X_ecef
  Gain : Gain  Gain=1.14*10e-7
  Gain1 : Gain  Gain=4*10e-7
  Position to VRML : $bdroot/Virtual World/Position to VRML  SystemSampleTime=-1  Latency=0  AutoFrameSizeCalculation=off
  Position to VRML1 : $bdroot/Virtual World/Position to VRML  SystemSampleTime=-1  Latency=0  AutoFrameSizeCalculation=off
  Quaternion to VRML : $bdroot/Virtual World/Quaternion to VRML  SystemSampleTime=-1  Latency=0  AutoFrameSizeCalculation=off
  Sun's Position to ECEF : $bdroot/Virtual World/Sun's Position to ECEF  SystemSampleTime=-1  Latency=0  AutoFrameSizeCalculation=off
  Sat Rot : Outport
  Sat Pos : Outport  Port=2
  Sun Pos : Outport  Port=3
  wires:
  Position to VRML1/1 -> Sun Pos/1
  Env/1 -> Sun's Position to ECEF/1
  SatStates/1 -> Bus Selector/1
  Gain/1 -> Position to VRML/1
  Bus Selector/1 -> Quaternion to VRML/1  "<q_ECEF2Body>"
  Bus Selector/2 -> Gain/1  "<X_ecef>"
  Quaternion to VRML/1 -> Sat Rot/1
  Gain1/1 -> Position to VRML1/1
  Sun's Position to ECEF/1 -> Gain1/1
  Position to VRML/1 -> Sat Pos/1

== system scarsLibrary/Virtual World/Sun's Position to ECEF ==
  note: Parametrise DCM
  Bus Element In : Inport  PortName=Env  Element=Sun's Position [km]
  Clock : Clock
  Direction Cosine Matrix ECI to ECEF : aerolibtransform2/Direction Cosine Matrix ECI to ECEF  red=IAU-2000/2006  year=2000  month=January  day=1  hour=12  min=0  sec=0  deltaT=Sec  errorflag=Error  extraparamflag=off
      settings: AttributesFormatString=%<red>  SourceProductName=Aerospace Blockset  SourceProductBaseCode=AE
  Direction Cosine Matrix to Quaternions : sharedtransform/Direction Cosine Matrix  to Quaternions  aMode=0  action=None  tolerance=eps(2)
      settings: SourceProductName=Aerospace Blockset  SourceProductBaseCode=AE
  Quaternion Rotation : aerolibutil/Quaternion Rotation
  pos : Outport
  wires:
  Direction Cosine Matrix ECI to ECEF/1 -> Direction Cosine Matrix to Quaternions/1
  Direction Cosine Matrix to Quaternions/1 -> Quaternion Rotation/1
  Clock/1 -> Direction Cosine Matrix ECI to ECEF/1
  Quaternion Rotation/1 -> pos/1
  Bus Element In/1 -> Quaternion Rotation/2

== system scarsLibrary/Actuators/Bang-Bang Thrusters/Thruster Pitch ==
  Torque : Inport
  Gain2 : Gain  Gain=-1
  Relay1 : Relay  OnSwitchValue=bb.a1  OffSwitchValue=bb.a0  OnOutputValue=bb.thrust
  Relay2 : Relay  OnSwitchValue=bb.a1  OffSwitchValue=bb.a0  OnOutputValue=-bb.thrust
  Scope1 : Scope  NumInputPorts=5
  Sum1 : Sum  Inputs=-|-
  Sum2 : Sum  Inputs=+|+
  Torque Out : Outport
  wires:
  Torque/1 -> Gain2/1, Relay1/1, Scope1/1  "pd"
  Relay1/1 -> Sum2/1, Scope1/4
  Gain2/1 -> Relay2/1, Scope1/2
  Sum2/1 -> Sum1/1, Scope1/5
  Relay2/1 -> Sum2/2, Scope1/3
  Sum1/1 -> Torque Out/1  "M"

== system scarsLibrary/Actuators/Bang-Bang Thrusters/Thruster Roll ==
  Torque : Inport
  Gain2 : Gain  Gain=-1
  Noise : simulink/Sources/Band-Limited White Noise  Cov=[0.1]  Ts=0.1  seed=[23341]
  Relay1 : Relay  OnSwitchValue=bb.a1  OffSwitchValue=bb.a0  OnOutputValue=bb.thrust
  Relay2 : Relay  OnSwitchValue=bb.a1  OffSwitchValue=bb.a0  OnOutputValue=-bb.thrust
  Sum2 : Sum  Inputs=+++
  Torque Out : Outport
  wires:
  Torque/1 -> Gain2/1, Relay1/1
  Relay1/1 -> Sum2/1
  Gain2/1 -> Relay2/1
  Sum2/1 -> Torque Out/1
  Relay2/1 -> Sum2/3
  Noise/1 -> Sum2/2

== system scarsLibrary/Actuators/Bang-Bang Thrusters/Thruster Yaw ==
  Torque : Inport
  Constant : Constant  Value=bb.a0
  Constant1 : Constant  Value=bb.a1
  Gain2 : Gain  Gain=-1
  Mux : Mux  Inputs=3
  Mux1 : Mux
  Relay1 : Relay  OnSwitchValue=bb.a1  OffSwitchValue=bb.a0  OnOutputValue=bb.thrust
  Relay2 : Relay  OnSwitchValue=bb.a1  OffSwitchValue=bb.a0  OnOutputValue=-bb.thrust
  Scope1 : Scope  NumInputPorts=2
  Sum1 : Sum  Inputs=-|-
  Sum2 : Sum  Inputs=+|+
  Torque Out : Outport
  wires:
  Constant1/1 -> Mux1/4
  Constant/1 -> Mux1/3
  Mux/1 -> Scope1/2
  Mux1/1 -> Scope1/1  "acutator cmd"
  Torque/1 -> Gain2/1, Mux1/1, Relay1/1  "Actuator Cmd"
  Relay1/1 -> Sum2/1, Mux/2  "Plus Relay"
  Gain2/1 -> Relay2/1, Mux1/2
  Sum2/1 -> Sum1/1, Mux/3  "M"
  Relay2/1 -> Sum2/2, Mux/1  "Minus Relay"
  Sum1/1 -> Torque Out/1  "M"

== system scarsLibrary/Actuators/Drag Sail/Drag  ==
  Bus Element In : Inport  PortName=SatStates  Element=V_B
  Bus Element In1 : Inport  PortName=SatStates  Element=Euler_B
  Density : Inport  Port=2
  Abs : Abs
  Add : Sum  Inputs=+++
  Constant1 : Constant  Value=area_vector
  Cos : Trigonometry  Operator=cos
  Demux : Demux  Outputs=3
  Gain : Gain  Gain=-1/2*C_d
  Normalize Vector : vrlib/Utilities/Normalize Vector  maxzero=0
      settings: SourceProductName=Simulink
  Product : Product  Inputs=3
  Product1 : Product
  Product2 : Product
  Quaternion Rotation : aerolibutil/Quaternion Rotation
  Rotation Angles to Quaternions : sharedtransform/Rotation Angles to Quaternions  rotationOrder=XYZ  aMode=aMode
      settings: SourceProductName=Aerospace Blockset  SourceProductBaseCode=AE
  Square : Math  Operator=square  SignedPower=off  SaturateOnIntegerOverflow=on
  Subsystem : $bdroot/Subsystem  SystemSampleTime=-1  Latency=0  AutoFrameSizeCalculation=off
  Vector Norm : $bdroot/Vector Norm  SystemSampleTime=-1  Latency=0  AutoFrameSizeCalculation=off
  Force : Outport
  wires:
  Gain/1 -> Product/2
  Product/1 -> Product1/2
  Product1/1 -> Force/1
  Normalize Vector/1 -> Product1/1
  Density/1 -> Product/3
  Bus Element In1/1 -> Rotation Angles to Quaternions/1
  Constant1/1 -> Product2/1
  Product2/1 -> Gain/1
  Rotation Angles to Quaternions/1 -> Quaternion Rotation/1
  Bus Element In/1 -> Vector Norm/1, Normalize Vector/1, Quaternion Rotation/2
  Quaternion Rotation/1 -> Subsystem/1
  Subsystem/1 -> Cos/1
  Demux/1 -> Add/1
  Demux/2 -> Add/2
  Demux/3 -> Add/3
  Cos/1 -> Abs/1
  Add/1 -> Product2/2
  Vector Norm/1 -> Square/1
  Square/1 -> Product/1
  Abs/1 -> Demux/1

== system scarsLibrary/Actuators/Drag Sail (1-axis)/Drag  ==
  Bus Element In : Inport  PortName=SatStates  Element=V_B
  Bus Element In1 : Inport  PortName=SatStates  Element=Euler_B
  Density : Inport  Port=2
  Abs : Abs
  Add : Sum  Inputs=+++
  Constant1 : Constant  Value=[A_x, A_y, A_z]
  Cos : Trigonometry  Operator=cos
  Demux : Demux  Outputs=3
  Gain : Gain  Gain=-1/2*C_d
  Normalize Vector : vrlib/Utilities/Normalize Vector  maxzero=0
      settings: SourceProductName=Simulink
  Product : Product  Inputs=3
  Product1 : Product
  Product2 : Product
  Quaternion Rotation : aerolibutil/Quaternion Rotation
  Rotation Angles to Quaternions : sharedtransform/Rotation Angles to Quaternions  rotationOrder=XYZ  aMode=aMode
      settings: SourceProductName=Aerospace Blockset  SourceProductBaseCode=AE
  Square : Math  Operator=square  SignedPower=off  SaturateOnIntegerOverflow=on
  Subsystem : $bdroot/Subsystem  SystemSampleTime=-1  Latency=0  AutoFrameSizeCalculation=off
  Vector Norm : $bdroot/Vector Norm  SystemSampleTime=-1  Latency=0  AutoFrameSizeCalculation=off
  Force : Outport
  wires:
  Abs/1 -> Demux/1
  Square/1 -> Product/1
  Vector Norm/1 -> Square/1
  Add/1 -> Product2/2
  Cos/1 -> Abs/1
  Demux/3 -> Add/3
  Demux/2 -> Add/2
  Demux/1 -> Add/1
  Subsystem/1 -> Cos/1
  Quaternion Rotation/1 -> Subsystem/1
  Bus Element In/1 -> Quaternion Rotation/2, Normalize Vector/1, Vector Norm/1
  Rotation Angles to Quaternions/1 -> Quaternion Rotation/1
  Product2/1 -> Gain/1
  Constant1/1 -> Product2/1
  Bus Element In1/1 -> Rotation Angles to Quaternions/1
  Density/1 -> Product/3
  Normalize Vector/1 -> Product1/1
  Product1/1 -> Force/1
  Product/1 -> Product1/2
  Gain/1 -> Product/2

== system scarsLibrary/Actuators/Reaction Wheels/Reaction Wheel Pitch ==
  note: Disturbances can
      | be put here
  note: input here
  note: qw - anqular velocity
      |  of the wheel
  Rate : Inport
  Torque : Inport  Port=2
  Gain : Gain  Gain=rw.N
  Gain1 : Gain  Gain=rw.N/rw.R
  Gain2 : Gain  Gain=-rw.c
  Integrator : Integrator
  Scope : Scope  NumInputPorts=2
  Sum : Sum  Inputs=+|-
  Sum1 : Sum  Inputs=+|+
  Sum2 : Sum  Inputs=+|-
  Sum3 : Sum  Inputs=-|-
  Transfer Fcn : TransferFcn  Denominator=[rw.J 0]
  Torque Out : Outport
  wires:
  Transfer Fcn/1 -> Sum2/2  "qw"
  Sum/1 -> Gain1/1  "Ri"
  Sum2/1 -> Gain2/1, Gain/1
  Rate/1 -> Scope/1, Integrator/1, Sum2/1  "q"
  Gain/1 -> Sum/2  "N(q_qw)"
  Sum1/1 -> Torque Out/1  "M:2"
  Torque/1 -> Sum/1  "e"
  Sum3/1 -> Transfer Fcn/1
  Integrator/1 -> Scope/2  "theta"
  Gain1/1 -> Sum3/1, Sum1/1  "Ni"
  Gain2/1 -> Sum3/2, Sum1/2  "Qf"

== system scarsLibrary/Actuators/Reaction Wheels/Reaction Wheel Roll ==
  note: qw - anqular velocity
      |  of the wheel
  note: input here
  note: Disturbances can
      | be put here
  Rate : Inport
  Torque : Inport  Port=2
  Gain : Gain  Gain=rw.N
  Gain1 : Gain  Gain=rw.N/rw.R
  Gain2 : Gain  Gain=-rw.c
  Integrator : Integrator
  Scope : Scope  NumInputPorts=2
  Sum : Sum  Inputs=+|-
  Sum1 : Sum  Inputs=+|+
  Sum2 : Sum  Inputs=+|-
  Sum3 : Sum  Inputs=-|-
  Transfer Fcn : TransferFcn  Denominator=[rw.J 0]
  Torque Out : Outport
  wires:
  Rate/1 -> Scope/1, Integrator/1, Sum2/1  "q"
  Gain/1 -> Sum/2  "N(q_qw)"
  Sum2/1 -> Gain/1, Gain2/1
  Sum1/1 -> Torque Out/1  "M:1"
  Gain2/1 -> Sum3/2, Sum1/2  "Qf"
  Transfer Fcn/1 -> Sum2/2  "qw"
  Integrator/1 -> Scope/2  "theta"
  Sum/1 -> Gain1/1  "Ri"
  Sum3/1 -> Transfer Fcn/1
  Torque/1 -> Sum/1  "e"
  Gain1/1 -> Sum3/1, Sum1/1  "Ni"

== system scarsLibrary/Actuators/Reaction Wheels/Reaction Wheel Yaw ==
  note: Disturbances can
      | be put here
  note: input here
  note: qw - anqular velocity
      |  of the wheel
  Rate : Inport
  Torque : Inport  Port=2
  Gain : Gain  Gain=rw.N
  Gain1 : Gain  Gain=rw.N/rw.R
  Gain2 : Gain  Gain=-rw.c
  Integrator : Integrator
  Scope : Scope  NumInputPorts=2
  Sum : Sum  Inputs=+|-
  Sum1 : Sum  Inputs=+|+
  Sum2 : Sum  Inputs=+|-
  Sum3 : Sum  Inputs=-|-
  Transfer Fcn : TransferFcn  Denominator=[rw.J 0]
  Torque Out : Outport
  wires:
  Transfer Fcn/1 -> Sum2/2  "qw"
  Sum/1 -> Gain1/1  "Ri"
  Sum2/1 -> Gain2/1, Gain/1
  Rate/1 -> Scope/1, Integrator/1, Sum2/1  "q"
  Gain/1 -> Sum/2  "N(q_qw)"
  Sum1/1 -> Torque Out/1  "M:3"
  Torque/1 -> Sum/1  "e"
  Sum3/1 -> Transfer Fcn/1
  Integrator/1 -> Scope/2  "theta"
  Gain1/1 -> Sum3/1, Sum1/1  "Ni"
  Gain2/1 -> Sum3/2, Sum1/2  "Qf"

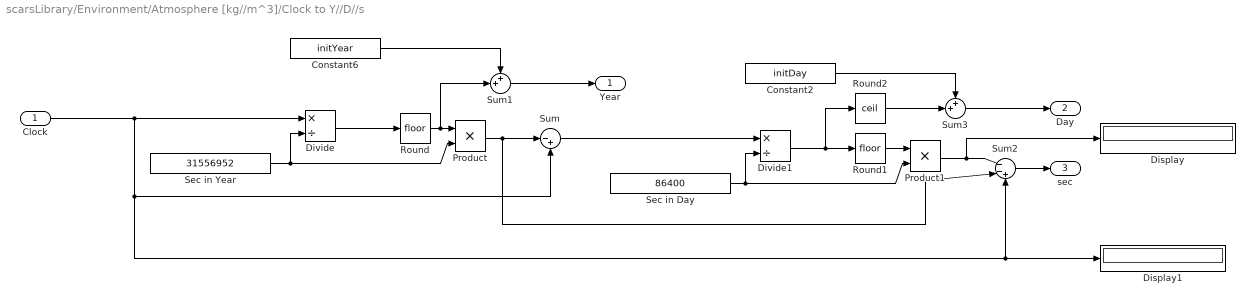
== system scarsLibrary/Environment/Atmosphere [kg//m^3]/Clock to Y//D//s ==
  Clock : Inport
  Constant2 : Constant  Value=initDay
  Constant6 : Constant  Value=initYear
  Display : Display
  Display1 : Display
  Divide : Product  Inputs=*/
  Divide1 : Product  Inputs=*/
  Product : Product
  Product1 : Product
  Round : Rounding
  Round1 : Rounding
  Round2 : Rounding  Operator=ceil
  Sec in Day : Constant  Value=86400
  Sec in Year : Constant  Value=31556952
  Sum : Sum  Inputs=|-+
  Sum1 : Sum  Inputs=++|
  Sum2 : Sum  Inputs=|--+
  Sum3 : Sum  Inputs=++|
  Year : Outport
  Day : Outport  Port=2
  sec : Outport  Port=3
  wires:
  Sum1/1 -> Year/1
  Sum3/1 -> Day/1
  Round1/1 -> Product1/1
  Sum2/1 -> sec/1
  Product/1 -> Sum2/2, Sum/1
  Round/1 -> Sum1/2, Product/1
  Sum/1 -> Divide1/1
  Divide1/1 -> Round2/1, Round1/1
  Product1/1 -> Display/1, Sum2/1
  Sec in Day/1 -> Product1/2, Divide1/2
  Constant2/1 -> Sum3/1
  Sec in Year/1 -> Product/2, Divide/2
  Divide/1 -> Round/1
  Clock/1 -> Divide/1, Sum2/3, Display1/1, Sum/2
  Constant6/1 -> Sum1/1
  Round2/1 -> Sum3/2

== system scarsLibrary/Environment/Magnetic Field [nT]/Magnetic Model ==
  DecimalYear : Inport
  Bus Element In : Inport  Port=2  PortName=SatStates  Element=lla
  Demux : Demux  Outputs=3
  Terminator{,1..3} (4 alike) : Terminator
  World Magnetic Model : aerolibgravity2/World Magnetic Model  model=WMM2015 V2 (2015-2020)  customFile='WMM2015v2.COF'  units=Metric (MKS)  time_in=on  month=January  day=1  year=2015  action=Error  h_out=on  dec_out=on  inc_out=on  ti_out=on
      settings: SourceProductName=Aerospace Blockset  SourceProductBaseCode=AE
  MagneticField : Outport
  wires:
  DecimalYear/1 -> World Magnetic Model/4
  World Magnetic Model/1 -> MagneticField/1
  World Magnetic Model/2 -> Terminator/1
  World Magnetic Model/5 -> Terminator3/1
  World Magnetic Model/3 -> Terminator1/1
  World Magnetic Model/4 -> Terminator2/1
  Demux/1 -> World Magnetic Model/2
  Demux/2 -> World Magnetic Model/3
  Demux/3 -> World Magnetic Model/1
  Bus Element In/1 -> Demux/1

== system scarsLibrary/Environment/Magnetic Field [nT]/Time2Decyear ==
  " " : Inport
  Decsec : Gain  Gain=decsec
  Initial Decyear : Constant  Value=decstart
  Sum : Sum  Inputs=|++
  "  " : Outport
  wires:
  Initial Decyear/1 -> Sum/1
  " "/1 -> Decsec/1
  Decsec/1 -> Sum/2
  Sum/1 -> "  "/1

== system scarsLibrary/PW-Sat2/Drag Sail/Drag  ==
  Bus Element In : Inport  PortName=SatStates  Element=V_B
  Bus Element In1 : Inport  PortName=SatStates  Element=Euler_B
  Density : Inport  Port=2
  Abs : Abs
  Add : Sum  Inputs=+++
  Constant1 : Constant  Value=area_vector
  Cos : Trigonometry  Operator=cos
  Demux : Demux  Outputs=3
  Gain : Gain  Gain=-1/2*C_d
  Normalize Vector : vrlib/Utilities/Normalize Vector  maxzero=0
      settings: SourceProductName=Simulink
  Product : Product  Inputs=3
  Product1 : Product
  Product2 : Product
  Quaternion Rotation : aerolibutil/Quaternion Rotation
  Rotation Angles to Quaternions : sharedtransform/Rotation Angles to Quaternions  rotationOrder=XYZ  aMode=aMode
      settings: SourceProductName=Aerospace Blockset  SourceProductBaseCode=AE
  Square : Math  Operator=square  SignedPower=off  SaturateOnIntegerOverflow=on
  Subsystem : $bdroot/Subsystem  SystemSampleTime=-1  Latency=0  AutoFrameSizeCalculation=off
  Vector Norm : $bdroot/Vector Norm  SystemSampleTime=-1  Latency=0  AutoFrameSizeCalculation=off
  Force : Outport
  wires:
  Abs/1 -> Demux/1
  Square/1 -> Product/1
  Vector Norm/1 -> Square/1
  Add/1 -> Product2/2
  Cos/1 -> Abs/1
  Demux/3 -> Add/3
  Demux/2 -> Add/2
  Demux/1 -> Add/1
  Subsystem/1 -> Cos/1
  Quaternion Rotation/1 -> Subsystem/1
  Bus Element In/1 -> Quaternion Rotation/2, Normalize Vector/1, Vector Norm/1
  Rotation Angles to Quaternions/1 -> Quaternion Rotation/1
  Product2/1 -> Gain/1
  Constant1/1 -> Product2/1
  Bus Element In1/1 -> Rotation Angles to Quaternions/1
  Density/1 -> Product/3
  Normalize Vector/1 -> Product1/1
  Product1/1 -> Force/1
  Product/1 -> Product1/2
  Gain/1 -> Product/2

== system scarsLibrary/Standard/Satellite Dynamics/Forces Switch ==
  In : Inport
  Constant1 : Constant  Value=[0 0 0]
  Forces : Constant
  Switch : Switch  Criteria=u2 > Threshold
  Out : Outport
  wires:
  Constant1/1 -> Switch/3
  Forces/1 -> Switch/2
  Switch/1 -> Out/1
  In/1 -> Switch/1

== system scarsLibrary/Standard/Satellite Dynamics/Moments Switch ==
  In : Inport
  Constant1 : Constant  Value=[0 0 0]
  Moments : Constant
  Switch : Switch  Criteria=u2 > Threshold
  Out : Outport
  wires:
  In/1 -> Switch/1
  Constant1/1 -> Switch/3
  Switch/1 -> Out/1
  Moments/1 -> Switch/2
